simulink model "hardstop"  (Simulink 6.0)
settings: Solver=ode45  SolverMode=SingleTasking  StartTime=0.0  StopTime=2.0  RelTol=1e-6  AbsTol=1e-6
settings Model: Creator=The MathWorks Inc.  LastModifiedBy=batserve  ExtModeTrigMode=oneshot  ExtModeArmWhenConnect=off  ExtModeAutoUpdateStatusClock=off
settings DataIOCC: ExternalInput=[]  InitialState=[]  LimitDataPoints=off  SaveFormat=StructureWithTime  SaveState=on
settings DebuggingCC: CheckExecutionContextPreStartOutputMsg=on  CheckExecutionContextRuntimeOutputMsg=on  SolverPrmCheckMsg=none  IntegerOverflowMsg=none
settings HardwareCC: TargetUnknown=on

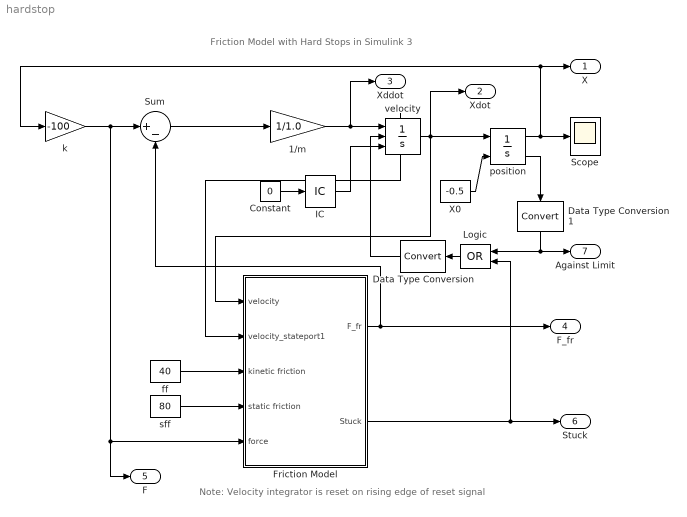
== system hardstop ==
  note: Friction Model with Hard Stops in Simulink 3
  note: Note: Velocity integrator is reset on rising edge of reset signal
  1/m : Gain  Gain=1/1.0  SaturateOnIntegerOverflow=on
  Constant : Constant  Value=0
  Data Type Conversion : DataTypeConversion  Orientation=left  OutDataTypeMode=double  SaturateOnIntegerOverflow=on  RndMeth=Zero
  Data Type Conversion1 : DataTypeConversion  Orientation=down  OutDataTypeMode=boolean  SaturateOnIntegerOverflow=on  RndMeth=Zero
  Friction Model : Subsystem  PropExecContextAcrossSSBoundary=on
  IC : InitialCondition  Value=100
  Logic : Logic  Orientation=left  Operator=OR
  Scope : Scope
      settings: TickLabels=on  YMin=-4  YMax=6  DataFormat=Array
  Sum : Sum  Inputs=|+-  SaturateOnIntegerOverflow=on  InputSameDT=on
  X0 : Constant  Value=-0.5
  ff : Constant  Value=40
  k : Gain  Gain=-100  SaturateOnIntegerOverflow=on
  position : Integrator  InitialConditionSource=external  LimitOutput=on  UpperSaturationLimit=5.5  LowerSaturationLimit=-3.5  ShowSaturationPort=on
  sff : Constant  Value=80
  velocity : Integrator  ExternalReset=rising  InitialConditionSource=external  ShowStatePort=on
  X : Outport  InitialOutput=0
  Xdot : Outport  Port=2  InitialOutput=0
  Xddot : Outport  Port=3  InitialOutput=0
  F_fr : Outport  Port=4  InitialOutput=0
  F : Outport  Port=5  InitialOutput=0
  Stuck : Outport  Port=6  InitialOutput=0
  Against Limit : Outport  Port=7  InitialOutput=0
  wires:
  position/1 -> Scope/1, k/1, X/1
  position/2 -> Data Type Conversion1/1
  Constant/1 -> IC/1
  X0/1 -> position/2
  Sum/1 -> 1/m/1
  IC/1 -> velocity/3
  velocity/1 -> Xdot/1, position/1, Friction Model/1(velocity)
  k/1 -> Sum/1, F/1, Friction Model/5(force)
  1/m/1 -> velocity/1, Xddot/1
  sff/1 -> Friction Model/4(static friction)
  ff/1 -> Friction Model/3(kinetic friction)
  Friction Model/2(Stuck) -> Stuck/1, Logic/2
  velocity/State -> Friction Model/2(velocity_stateport1)
  Logic/1 -> Data Type Conversion/1
  Friction Model/1(F_fr) -> F_fr/1, Sum/2
  Data Type Conversion/1 -> velocity/2
  Data Type Conversion1/1 -> Against Limit/1, Logic/1

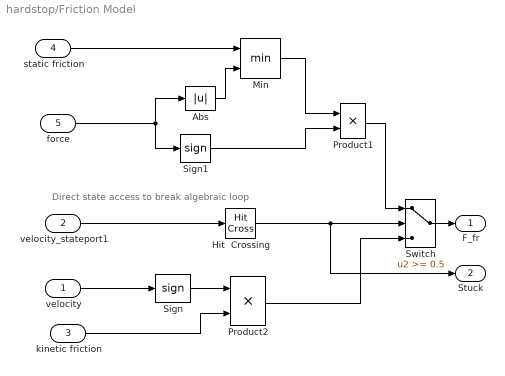
== system hardstop/Friction Model ==
  note: Direct state access to
      | break algebraic loop
  velocity : Inport  Port=1  LatchInput=off
  velocity_stateport1 : Inport  Port=2  LatchInput=off
  kinetic friction : Inport  Port=3  LatchInput=off
  static friction : Inport  Port=4  LatchInput=off
  force : Inport  Port=5  LatchInput=off
  Abs : Abs  SaturateOnIntegerOverflow=on
  Hit  Crossing : HitCross
  Min : MinMax  Inputs=2  SaturateOnIntegerOverflow=on  InputSameDT=on
  Product1 : Product  SaturateOnIntegerOverflow=on  InputSameDT=on
  Product2 : Product  SaturateOnIntegerOverflow=on  InputSameDT=on
  Sign : Signum
  Sign1 : Signum
  Switch : Switch  Threshold=0.5  SaturateOnIntegerOverflow=on  InputSameDT=on
  F_fr : Outport  InitialOutput=0
  Stuck : Outport  Port=2  InitialOutput=0
  wires:
  Hit  Crossing/1 -> Stuck/1, Switch/2
  Product2/1 -> Switch/3
  kinetic friction/1 -> Product2/2
  Sign/1 -> Product2/1
  velocity/1 -> Sign/1
  Switch/1 -> F_fr/1
  velocity_stateport1/1 -> Hit  Crossing/1
  Product1/1 -> Switch/1
  force/1 -> Abs/1, Sign1/1
  Abs/1 -> Min/2
  static friction/1 -> Min/1
  Min/1 -> Product1/1
  Sign1/1 -> Product1/2
